simulink model "example"  (R2024a)
settings: Solver=FixedStepAuto  StartTime=0.0  StopTime=2  FixedStep=0.001  RelTol=1e-3  EnableMultiTasking=on
settings Model: Param_HCUVersion=EAXVA04V2MCU  Creator=yanaolangde  LastModifiedBy=autod
settings DataIOCC: SaveFormat=Structure  SignalLoggingSaveFormat=ModelDataLogs  SaveOutput=off  SignalLogging=off  DSMLogging=off  SaveTime=off  ReturnWorkspaceOutputs=off
settings OptimizationCC: DefaultParameterBehavior=Inlined  InlineInvariantSignals=on  EnhancedBackFolding=on  EnableMemcpy=off  PassReuseOutputArgsAs=Individual arguments  ZeroExternalMemoryAtStartup=off  ZeroInternalMemoryAtStartup=off  EfficientFloat2IntCast=on  SimCompilerOptimization=on  OptimizeBlockOrder=speed  DifferentSizesBufferReuse=on  EfficientTunableParamExpr=on
settings DebuggingCC: AlgebraicLoopMsg=none  ArtificialAlgebraicLoopMsg=none  SaveWithDisabledLinksMsg=none  SaveWithParameterizedLinksMsg=none  CheckSSInitialOutputMsg=off  UnderspecifiedInitializationDetection=Classic  SignalResolutionControl=TryResolveAll  BlockPriorityViolationMsg=error  MinStepSizeMsg=none  InheritedTsInSrcMsg=none  MultiTaskDSMMsg=none  MultiTaskCondExecSysMsg=none  MultiTaskRateTransMsg=warning  TasksWithSamePriorityMsg=none  SigSpecEnsureSampleTimeMsg=none  Int32ToFloatConvMsg=none  ParameterPrecisionLossMsg=none  ParameterTunabilityLossMsg=error  FixptConstOverflowMsg=error  FcnCallInpInsideContextMsg=warning  UnconnectedInputMsg=error  UnconnectedOutputMsg=error  UnconnectedLineMsg=error  FrameProcessingCompatibilityMsg=none  BusObjectLabelMismatch=none  RootOutportRequireBusObject=none  UnknownTsInhSupMsg=none  ModelReferenceDataLoggingMessage=none  OperatingPointInterfaceChecksumMismatchMsg=none  SFUnusedDataAndEventsDiag=none  SFUnexpectedBacktrackingDiag=none  SFInvalidInputDataAccessInChartInitDiag=none  SFNoUnconditionalDefaultTransitionDiag=none  SFTransitionOutsideNaturalParentDiag=none  SFUnreachableExecutionPathDiag=none
settings HardwareCC: ProdBitPerPointer=32  ProdBitPerSizeT=32  ProdBitPerPtrDiffT=32  ProdLargestAtomicFloat=None  ProdWordSize=32  ProdLongLongMode=on  ProdHWDeviceType=Infineon->TriCore
settings ModelReferenceCC: UpdateModelReferenceTargets=Force  PropagateSignalLabelsOutOfModel=off
settings SFSimCC: SFSimEcho=off  MATLABDynamicMemAlloc=off
settings RTWCC: Description=Ecotrons TC2xx  SystemTargetFile=EcoCoderTC27x.tlc  GenerateMakefile=off  TemplateMakefile=ert_default_tmf  RTWVerbose=off  RetainRTWFile=on  RTWCompilerOptimization=on  GPUComputeCapability=3.5
settings CodeAppCC: IgnoreCustomStorageClasses=off  OperatorAnnotations=on  CustomSymbolStrGlobalVar=$N$M  CustomSymbolStrType=$N$M  CustomSymbolStrFcn=$N$M  CustomSymbolStrFcnArg=$N$M  CustomSymbolStrBlkIO=$N$M  CustomSymbolStrMacro=$N$M
settings STFCustomTargetCC: CodeReplacementLibrary=ANSI_C  MultiwordLength=256  IncludeMdlTerminateFcn=off  CombineOutputUpdateFcns=on  SuppressErrorStatus=on  ERTCustomFileBanners=on  SupportNonFinite=off  SupportComplex=off  SupportContinuousTime=off  SupportNonInlinedSFcns=off  RemoveResetFunc=on  MATLABClassNameForMDSCustomization=Simulink.SoftwareTarget.ERTCustomization  GRTInterface=off  UseToolchainInfoCompliant=off  SystemTargetFile=EcoCoderTC27x.tlc
settings ERTTargetCC: TargetLangStandard=C99 (ISO)  CodeReplacementLibrary=ANSI_C  ParMdlRefBuildCompliant=off  CompOptLevelCompliant=off  ConcurrentExecutionCompliant=off  IncludeMdlTerminateFcn=off  SuppressErrorStatus=on  SupportNonFinite=off  SupportComplex=off  ModelStepFunctionPrototypeControlCompliant=off  CPPClassGenCompliant=off  UseToolchainInfoCompliant=off  InlinedParameterPlacement=NonHierarchical  ERTCustomFileTemplate=example_file_process.tlc

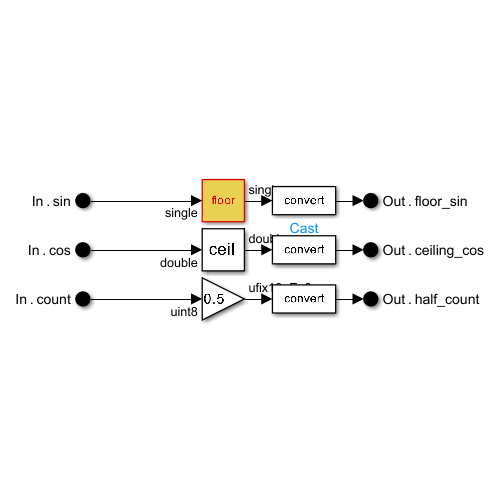
[thumbnail: Simulink's stored preview of the top-level diagram]
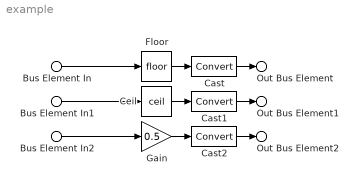
== system example ==
  Bus Element In : Inport  PortName=In  Element=sin
  Bus Element In1 : Inport  PortName=In  Element=cos
  Bus Element In2 : Inport  PortName=In  Element=count
  Cast : DataTypeConversion  SaturateOnIntegerOverflow=off  RndMeth=Floor
  Cast1 : DataTypeConversion  SaturateOnIntegerOverflow=off  RndMeth=Floor
  Cast2 : DataTypeConversion  SaturateOnIntegerOverflow=off  RndMeth=Floor
  Ceil : Rounding  Operator=ceil
  Floor : Rounding
  Gain : Gain  Gain=0.5
  Out Bus Element : Outport  PortName=Out  Element=floor_sin
  Out Bus Element1 : Outport  PortName=Out  Element=ceiling_cos
  Out Bus Element2 : Outport  PortName=Out  Element=half_count
  wires:
  Bus Element In/1 -> Floor/1
  Floor/1 -> Cast/1
  Bus Element In1/1 -> Ceil/1
  Ceil/1 -> Cast1/1
  Bus Element In2/1 -> Gain/1
  Gain/1 -> Cast2/1
  Cast/1 -> Out Bus Element/1
  Cast1/1 -> Out Bus Element1/1
  Cast2/1 -> Out Bus Element2/1
